simulink model "downcounter"  (R2017b)
settings: Solver=VariableStepAuto  StartTime=0.0  StopTime=10.0  RelTol=1e-3
settings Model: Creator=BCAYR5W  LastModifiedBy=BCAYR5W

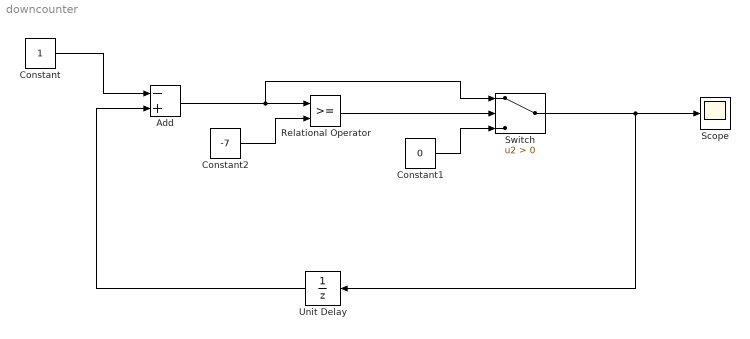
== system downcounter ==
  Add : Sum  Inputs=-+
  Constant : Constant
  Constant1 : Constant  Value=0
  Constant2 : Constant  Value=-7
  Relational Operator : RelationalOperator  OutDataTypeStr=boolean  RndMeth=Simplest
  Scope : Scope
  Switch : Switch  Criteria=u2 > Threshold
  Unit Delay : UnitDelay  InitialCondition=1  SampleTime=-1
  wires:
  Unit Delay/1 -> Add/2
  Constant2/1 -> Relational Operator/2
  Constant1/1 -> Switch/3
  Add/1 -> Switch/1, Relational Operator/1
  Constant/1 -> Add/1
  Relational Operator/1 -> Switch/2
  Switch/1 -> Scope/1, Unit Delay/1
